simulink model "simulinktrianguloypulso"  (R2015a)
settings: Solver=ode4  StartTime=-2.5  StopTime=2.5  FixedStep=1/100  RelTol=1e-3
libraries: simulink x3
settings Model: Creator=HP  LastModifiedBy=HP

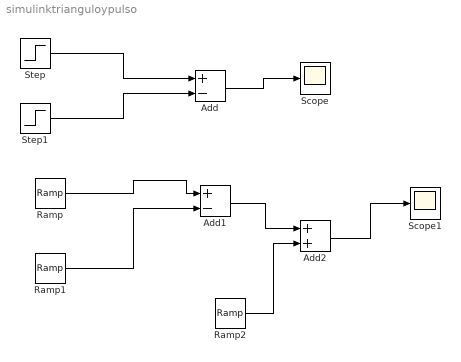
== system simulinktrianguloypulso ==
  Add : Sum  Inputs=+-
  Add1 : Sum  Inputs=+-
  Add2 : Sum
  Ramp : simulink/Sources/Ramp  slope=1  start=-1  X0=0
  Ramp1 : simulink/Sources/Ramp  slope=2  start=0  X0=0
  Ramp2 : simulink/Sources/Ramp  slope=1  start=1  X0=0
  Scope : Scope
      settings: SaveName=sumasteps
  Scope1 : Scope
      settings: SaveName=rampasuma
  Step : Step  Time=-1  SampleTime=0
  Step1 : Step  SampleTime=0
  wires:
  Step1/1 -> Add/2
  Step/1 -> Add/1
  Add/1 -> Scope/1
  Ramp/1 -> Add1/1
  Ramp1/1 -> Add1/2
  Add1/1 -> Add2/1
  Ramp2/1 -> Add2/2
  Add2/1 -> Scope1/1
